simulink model "starshipAltitudeControllerXplane"  (R2022a)
settings: Solver=VariableStepAuto  StartTime=0.0  StopTime=10.0  RelTol=1e-3
libraries: etargetslib x1, sldrtlib x1, dspnetwork x1
settings Model: Creator=Ammar Abdurrauf  LastModifiedBy=Ammar Abdurrauf

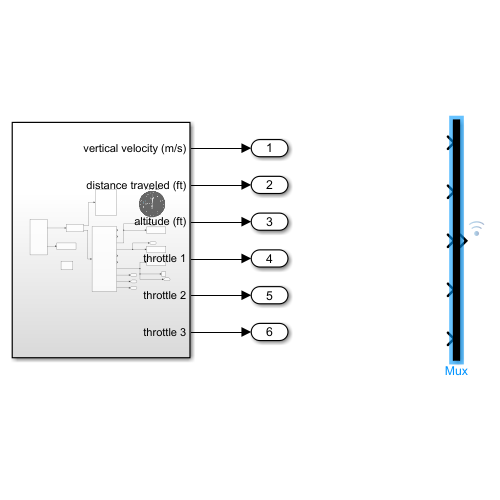
[thumbnail: Simulink's stored preview of the top-level diagram]
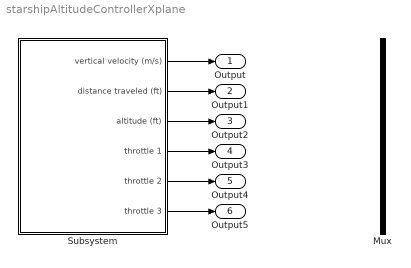
== system starshipAltitudeControllerXplane ==
  Mux : Mux  Inputs=5
  Subsystem : Subsystem
  Output : Outport
  Output1 : Outport  Port=2
  Output2 : Outport  Port=3
  Output3 : Outport  Port=4
  Output4 : Outport  Port=5
  Output5 : Outport  Port=6
  wires:
  Subsystem/1(vertical velocity (m/s)) -> Output/1
  Subsystem/2(distance traveled (ft)) -> Output1/1
  Subsystem/4(throttle 1) -> Output3/1
  Subsystem/3(altitude (ft)) -> Output2/1
  Subsystem/5(throttle 2) -> Output4/1
  Subsystem/6(throttle 3) -> Output5/1

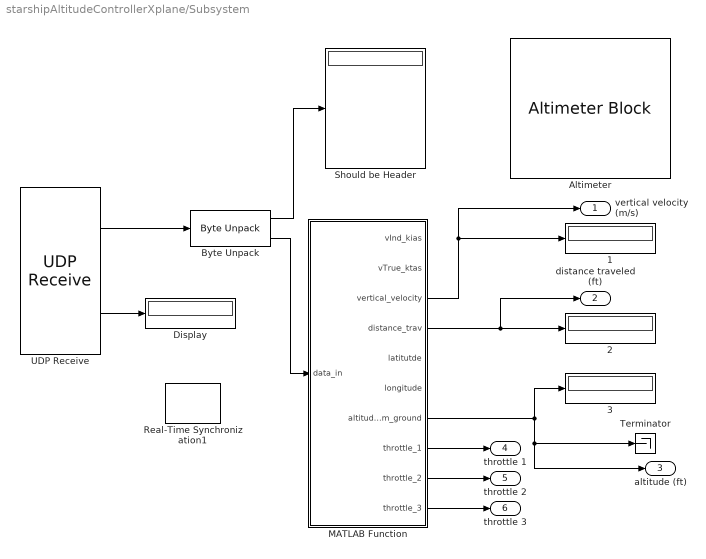
== system starshipAltitudeControllerXplane/Subsystem ==
  1 : Display
  2 : Display
  3 : Display
  Altimeter : AltimeterBlock
  Byte Unpack : etargetslib/Byte Unpack  dimensions={5,[9,8]}  datatypes={'uint8','single'}  byteAlign=1
  Display : Display
  MATLAB Function : MATLAB Function  TreatAsAtomicUnit=on
  Real-Time Synchronization1 : sldrtlib/Real-Time Synchronization  SampleTime=0.000235  MaxMissedTicks=100  ShowMissedTicks=off  YieldWhenWaiting=off
  Should be Header : Display
  Terminator : Terminator
  UDP Receive : dspnetwork/UDP Receive  localURL='0.0.0.0'  localPort=49004  remoteURL='127.0.0.1'  remotePort=-1  recvBufferSize=8192  dims=293  signalDatatype=uint8  isComplex=off  isVarSize=off  showBlockingTime=off  blockingTime=0  sampletime=0.000235  blockPlatform=[]
  vertical velocity (m/s) : Outport
  distance traveled (ft) : Outport  Port=2
  altitude (ft) : Outport  Port=3
  throttle 1 : Outport  Port=4
  throttle 2 : Outport  Port=5
  throttle 3 : Outport  Port=6
  wires:
  MATLAB Function/10(throttle_3) -> throttle 3/1
  MATLAB Function/7(altitude_from_ground) -> altitude (ft)/1, Terminator/1, 3/1
  MATLAB Function/8(throttle_1) -> throttle 1/1
  UDP Receive/1 -> Byte Unpack/1
  MATLAB Function/3(vertical_velocity) -> vertical velocity (m/s)/1, 1/1
  Byte Unpack/1 -> Should be Header/1
  MATLAB Function/4(distance_trav) -> distance traveled (ft)/1, 2/1
  UDP Receive/2 -> Display/1
  Byte Unpack/2 -> MATLAB Function/1(data_in)
  MATLAB Function/9(throttle_2) -> throttle 2/1

== matlab function starshipAltitudeControllerXplane/Subsystem/MATLAB Function ==
  data: data_in input; vInd_kias output; vTrue_ktas output; vertical_velocity output; distance_trav output; latitutde output; longitude output; altitude_from_ground output; throttle_1 output; throttle_2 output; throttle_3 output
function [vInd_kias,vTrue_ktas,...
    vertical_velocity, distance_trav,...
    latitutde, longitude, altitude_from_ground,...
    throttle_1, throttle_2, throttle_3] = decoder(data_in)
 
 vInd_kias = data_in(2,1);
 vTrue_ktas = data_in(4,1);
 latitutde= data_in(2,2);
 longitude= data_in(3,2);
 altitude_from_ground= data_in(5,2);
 vertical_velocity= data_in(6,3);
 distance_trav= data_in(8,3);
 throttle_1 = data_in(2, 4);
 throttle_2 = data_in(3, 4);
 throttle_3 = data_in(4, 4);
end
